simulink model "xi3_flatness"  (R2017b)
settings: Solver=VariableStepAuto  StartTime=0.0  StopTime=18  RelTol=1e-12
libraries: simulink x1
settings Model: Creator=chenjiasheng  LastModifiedBy=chenjiasheng

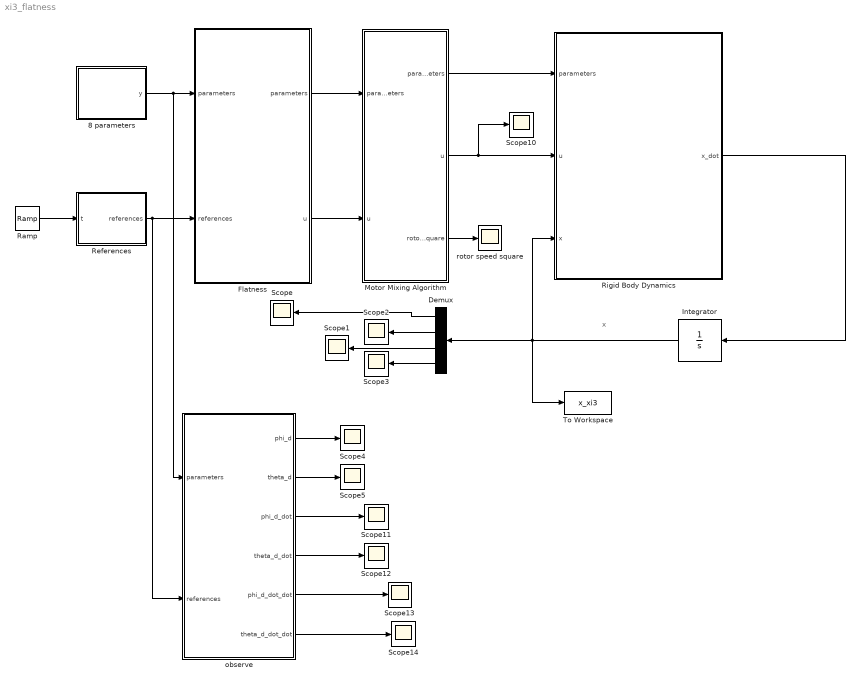
== system xi3_flatness ==
  note: x
  8 parameters : MATLAB Function  TreatAsAtomicUnit=on
  Demux : Demux
  Flatness : MATLAB Function  TreatAsAtomicUnit=on
  Integrator : Integrator  InitialCondition=x_xi2(end,:)  ContinuousStateAttributes='x'
  Motor Mixing Algorithm : MATLAB Function  TreatAsAtomicUnit=on
  Ramp : simulink/Sources/Ramp  slope=1  start=0  X0=0
  References : MATLAB Function  TreatAsAtomicUnit=on
  Rigid Body Dynamics : MATLAB Function  TreatAsAtomicUnit=on
  Scope{,1..5,10..14} (11 alike) : Scope
  To Workspace : ToWorkspace  VariableName=x_xi3  SampleTime=0.01
  observe : MATLAB Function  TreatAsAtomicUnit=on
  rotor speed square : Scope
  wires:
  Rigid Body Dynamics/1(x_dot) -> Integrator/1
  Motor Mixing Algorithm/3(rotor_speed_square) -> rotor speed square/1
  Motor Mixing Algorithm/1(parameters) -> Rigid Body Dynamics/1(parameters)
  Integrator/1 -> To Workspace/1, Demux/1, Rigid Body Dynamics/3(x)
  Motor Mixing Algorithm/2(u) -> Scope10/1, Rigid Body Dynamics/2(u)
  Ramp/1 -> References/1(t)
  Flatness/1(parameters) -> Motor Mixing Algorithm/1("parameters ")
  Flatness/2(u) -> Motor Mixing Algorithm/2("u ")
  References/1(references) -> Flatness/2(references), observe/2(references)
  8 parameters/1(y) -> Flatness/1("parameters "), observe/1(parameters)
  Demux/1 -> Scope/1
  Demux/3 -> Scope1/1
  Demux/2 -> Scope2/1
  Demux/4 -> Scope3/1
  observe/3(phi_d_dot) -> Scope11/1
  observe/4(theta_d_dot) -> Scope12/1
  observe/5(phi_d_dot_dot) -> Scope13/1
  observe/6(theta_d_dot_dot) -> Scope14/1
  observe/1(phi_d) -> Scope4/1
  observe/2(theta_d) -> Scope5/1

== matlab function xi3_flatness/Flatness ==
  data: parameters input; parameters output; references input; u output
function [parameters, u] = fcn(parameters,references)
% allocate input
m=parameters(1);
g=parameters(2);
M=diag(parameters(3:5));
r_d=references(1:3) ;          % reference's positions
r_d_dot=references(4:6);       % reference's velocities
a_d=references(7:9) ;          % reference's accelerations
a_d_dot=references(10:12);     % jerk
a_d_dot_dot=references(13:15); % snap
psi_d=references(16);          % reference's yaw angle 
psi_d_dot=references(17);
psi_d_dot_dot=references(18);

%% define some variables to make your life easier (f is not artifically defined)
f=m*sqrt(a_d(1)^2+a_d(2)^2+(g+a_d(3))^2);    % f is  the 1st element of input u
C=a_d(1)*cos(psi_d)+a_d(2)*sin(psi_d);      %
D=g+a_d(3);                                 %
A=a_d(1)*sin(psi_d)-a_d(2)*cos(psi_d);      %
B=sqrt(C^2+D^2);                            %
A_dot=sin(psi_d)*a_d_dot(1)-cos(psi_d)*a_d_dot(2)+C*psi_d_dot;                                   %
C_dot=cos(psi_d)*a_d_dot(1)+sin(psi_d)*a_d_dot(2)-A*psi_d_dot;                                   %
D_dot=a_d_dot(3);                                                                                %
B_dot=(C*C_dot+D*D_dot)/B;  
fbmsd=2*a_d(1)*a_d_dot(1)+2*a_d(2)*a_d_dot(2)+2*(g+a_d(3))*a_d_dot(3);   % f by m square dot
%% phi_d, theta_d
phi_d=asin(A*m/f) ;
if C>0
theta_d=acos(D/B) ;
else
theta_d=-acos(D/B) ;
end
%% phi_d_dot, theta_d_dot
phi_d_dot=(sin(psi_d)*(f/m)^2-A*a_d(1))/((f/m)^2*B)*a_d_dot(1) + (-cos(psi_d)*(f/m)^2-A*a_d(2))/((f/m)^2*B)*a_d_dot(2) + (-A*D)/((f/m)^2*B)*a_d_dot(3) + C/B*psi_d_dot;
theta_d_dot=(cos(psi_d)*D*a_d_dot(1)+sin(psi_d)*D*a_d_dot(2)-C*a_d_dot(3)-A*D*psi_d_dot)/B^2   ;

%% phi_d_dot_dot, theta_d_dot_dot
monster11=(cos(psi_d)*psi_d_dot*(f/m)^2+sin(psi_d)*fbmsd-(A_dot*a_d(1)+A*a_d_dot(1)))*a_d_dot(1)+(sin(psi_d)*(f/m)^2-A*a_d(1))*a_d_dot_dot(1);
monster12=(-sin(psi_d)*psi_d_dot*(f/m)^2+cos(psi_d)*fbmsd+A_dot*a_d(2)+A*a_d_dot(2))*a_d_dot(2)+(cos(psi_d)*(f/m)^2+A*a_d(2))*a_d_dot_dot(2);
monster13=(A_dot*D+A*D_dot)*a_d_dot(3)+A*D*a_d_dot_dot(3);
monster1=monster11-monster12-monster13;
phi_d_dot_dot=(monster1-(B*phi_d_dot-C*psi_d_dot)*fbmsd)/((f/m)^2*B) + (C_dot*psi_d_dot+C*psi_d_dot_dot-B_dot*phi_d_dot)/B;
monster21=(-sin(psi_d)*psi_d_dot*D+cos(psi_d)*D_dot)*a_d_dot(1)+cos(psi_d)*D*a_d_dot_dot(1);
monster22=(cos(psi_d)*psi_d_dot*D+sin(psi_d)*D_dot)*a_d_dot(2)+sin(psi_d)*D*a_d_dot_dot(2);
monster23= C_dot*a_d_dot(3)+C*a_d_dot_dot(3);
monster24=(A_dot*D+A*D_dot)*psi_d_dot+A*D*psi_d_dot_dot;
monster2= monster21+monster22-monster23-monster24;
theta_d_dot_dot=monster2/B^2-2*theta_d_dot*B_dot/B;

%% omegab, omegab_dot
Lnb=[1 0           -sin(theta_d);
     0 cos(phi_d)  sin(phi_d)*cos(theta_d);
     0 -sin(phi_d) cos(phi_d)*cos(theta_d)];
omegab=Lnb*[phi_d_dot;theta_d_dot;psi_d_dot];
omegab_dot=Lnb*[phi_d_dot_dot;theta_d_dot_dot;psi_d_dot_dot]+[-cos(theta_d)            0                        0;
                                                              -sin(phi_d)*sin(theta_d) cos(phi_d)*cos(theta_d)  -sin(phi_d);
                                                              -cos(phi_d)*sin(theta_d) -sin(phi_d)*cos(theta_d) -cos(phi_d)]*[theta_d_dot*psi_d_dot;phi_d_dot*psi_d_dot;phi_d_dot*theta_d_dot];

%% taub,u
taub=M*omegab_dot+cross(omegab,M*omegab);
u=[f;taub];
end

== matlab function xi3_flatness/8 parameters ==
  data: y output size=8
function y=fcn
%% specify parameters
m=0.468;
g=9.81;
Ix=4.856*10^(-3);
Iy=4.856*10^(-3);
Iz=8.801*10^(-3);
l=0.225;
k=2.980*10^-6;
c=1.140*10^-7;
%% output
y=[m;g;Ix;Iy;Iz;l;k;c] ;% output # 1-8
    
end

== matlab function xi3_flatness/observe ==
  data: parameters input; phi_d output; references input; theta_d output; phi_d_dot output; theta_d_dot output; phi_d_dot_dot output; theta_d_dot_dot output
function [phi_d,theta_d,phi_d_dot,theta_d_dot,phi_d_dot_dot,theta_d_dot_dot] = fcn(parameters,references)
% allocate input
m=parameters(1);
g=parameters(2);
M=diag(parameters(3:5));
r_d=references(1:3) ;          % reference's positions
r_d_dot=references(4:6);       % reference's velocities
a_d=references(7:9) ;          % reference's accelerations
a_d_dot=references(10:12);     % jerk
a_d_dot_dot=references(13:15); % snap
psi_d=references(16);          % reference's yaw angle 
psi_d_dot=references(17);
psi_d_dot_dot=references(18);

%% define some variables to make your life easier (f is not artifically defined)
f=m*sqrt(a_d(1)^2+a_d(2)^2+(g+a_d(3))^2);    % f is  the 1st element of input u
C=a_d(1)*cos(psi_d)+a_d(2)*sin(psi_d);      %
D=g+a_d(3);                                 %
A=a_d(1)*sin(psi_d)-a_d(2)*cos(psi_d);      %
B=sqrt(C^2+D^2);                            %
A_dot=sin(psi_d)*a_d_dot(1)-cos(psi_d)*a_d_dot(2)+C*psi_d_dot;                                   %   
C_dot=cos(psi_d)*a_d_dot(1)+sin(psi_d)*a_d_dot(2)-A*psi_d_dot;                                   %
D_dot=a_d_dot(3);                                                                                %
B_dot=(C*C_dot+D*D_dot)/B;
fbmsd=2*a_d(1)*a_d_dot(1)+2*a_d(2)*a_d_dot(2)+2*(g+a_d(3))*a_d_dot(3);   % f by m square dot
%% phi_d, theta_d
phi_d=asin(A*m/f) ;
if C>0
theta_d=acos(D/B) ;
else
theta_d=-acos(D/B) ;
end
%% phi_d_dot, theta_d_dot
phi_d_dot=(sin(psi_d)*(f/m)^2-A*a_d(1))/((f/m)^2*B)*a_d_dot(1) + (-cos(psi_d)*(f/m)^2-A*a_d(2))/((f/m)^2*B)*a_d_dot(2) + (-A*D)/((f/m)^2*B)*a_d_dot(3) + C/B*psi_d_dot;
theta_d_dot=(cos(psi_d)*D*a_d_dot(1)+sin(psi_d)*D*a_d_dot(2)-C*a_d_dot(3)-A*D*psi_d_dot)/B^2   ;

%% phi_d_dot_dot, theta_d_dot_dot
monster11=(cos(psi_d)*psi_d_dot*(f/m)^2+sin(psi_d)*fbmsd-(A_dot*a_d(1)+A*a_d_dot(1)))*a_d_dot(1)+(sin(psi_d)*(f/m)^2-A*a_d(1))*a_d_dot_dot(1);
monster12=(-sin(psi_d)*psi_d_dot*(f/m)^2+cos(psi_d)*fbmsd+A_dot*a_d(2)+A*a_d_dot(2))*a_d_dot(2)+(cos(psi_d)*(f/m)^2+A*a_d(2))*a_d_dot_dot(2);
monster13=(A_dot*D+A*D_dot)*a_d_dot(3)+A*D*a_d_dot_dot(3);
monster1=monster11-monster12-monster13;
phi_d_dot_dot=(monster1-(B*phi_d_dot-C*psi_d_dot)*fbmsd)/((f/m)^2*B) + (C_dot*psi_d_dot+C*psi_d_dot_dot-B_dot*phi_d_dot)/B;
monster21=(-sin(psi_d)*psi_d_dot*D+cos(psi_d)*D_dot)*a_d_dot(1)+cos(psi_d)*D*a_d_dot_dot(1);
monster22=(cos(psi_d)*psi_d_dot*D+sin(psi_d)*D_dot)*a_d_dot(2)+sin(psi_d)*D*a_d_dot_dot(2);
monster23= C_dot*a_d_dot(3)+C*a_d_dot_dot(3);
monster24=(A_dot*D+A*D_dot)*psi_d_dot+A*D*psi_d_dot_dot;
monster2= monster21+monster22-monster23-monster24;
theta_d_dot_dot=monster2/B^2-2*theta_d_dot*B_dot/B;

%% omegab, omegab_dot
Lnb=[1 0           -sin(theta_d);
     0 cos(phi_d)  sin(phi_d)*cos(theta_d);
     0 -sin(phi_d) cos(phi_d)*cos(theta_d)];
omegab=Lnb*[phi_d_dot;theta_d_dot;psi_d_dot];
omegab_dot=Lnb*[phi_d_dot_dot;theta_d_dot_dot;psi_d_dot_dot]+[-cos(theta_d)            0                        0;
                                                              -sin(phi_d)*sin(theta_d) cos(phi_d)*cos(theta_d)  -sin(phi_d);
                                                              -cos(phi_d)*sin(theta_d) -sin(phi_d)*cos(theta_d) -cos(phi_d)]*[theta_d_dot*psi_d_dot;phi_d_dot*psi_d_dot;phi_d_dot*theta_d_dot];

%% taub,u
taub=M*omegab_dot+cross(omegab,M*omegab);
u=[f;taub];
end

== matlab function xi3_flatness/References ==
  data: t input; references output size=18
function references = fcn(t)
%% specify your references here
g=9.81;
if t>=0 && t<2
r_desired=[0 0 0]'    ;              % reference's positions is not solved here
r_desired_dot=[0 0 0]'    ;          % reference's velocities is not solved here
r_desired_dot_dot=[0 0 0]'   ;       % reference's accelerations
r_desired_dot_dot_dot=[0 0 0]';      % jerk
r_desired_dot_dot_dot_dot=[0 0 0]' ; % snap
if t>=0 && t<1
psi_desired=pi/2-pi/4*t^2 ;                      % reference's yaw angle
psi_desired_dot=-pi/2*t;                  % reference's change rate of yaw angle       
psi_desired_dot_dot=-pi/2; 
else % t>=1 & t<2
psi_desired=pi/4*(t-2)^2 ;                      % reference's yaw angle
psi_desired_dot=pi/2*(t-2);                  % reference's change rate of yaw angle       
psi_desired_dot_dot=pi/2; 
end

elseif t>=2 && t<4  
if t>=2 && t<3
 r_desired=[0 0 0]'    ;              % reference's positions not solved here
 r_desired_dot=[0 0 0]'    ;          % reference's velocities not solved here
 r_desired_dot_dot=[0 0 -1]'   ;       % reference's accelerations
 r_desired_dot_dot_dot=[0 0 0]';      % jerk
 r_desired_dot_dot_dot_dot=[0 0 0]' ; % snap
else
 r_desired=[0 0 0]'    ;              % reference's positions 
 r_desired_dot=[0 0 0]'    ;          % reference's velocities 
 r_desired_dot_dot=[0 0 1]'   ;       % reference's accelerations
 r_desired_dot_dot_dot=[0 0 0]';      % jerk
 r_desired_dot_dot_dot_dot=[0 0 0]' ; % snap
end
 psi_desired=0 ;                      % reference's yaw angle
 psi_desired_dot=0 ;                  % reference's change rate of yaw angle       
 psi_desired_dot_dot=0;  
 
elseif t>=4 && t<6
tanalpha=0 ; % slope
if t>=4 && t<5
   [ax_d, az_d, ax_d_dot, az_d_dot, ax_d_dot_dot, az_d_dot_dot]=nest(t-4);
    ax_d=5/4*ax_d;                   az_d=5/4*az_d;
    ax_d_dot=5/4*ax_d_dot;           az_d_dot=5/4*az_d_dot;
    ax_d_dot_dot=5/4*ax_d_dot_dot;   az_d_dot_dot=5/4*az_d_dot_dot;
else % t>=5 && t<6
   [ax_d, az_d, ax_d_dot, az_d_dot, ax_d_dot_dot, az_d_dot_dot]=nest(t-5);
  ax_d=-5/4*ax_d;                 az_d=-5/4*az_d; % invert the direction for the sake of making end velocity zero
  ax_d_dot=-5/4*ax_d_dot;         az_d_dot=-5/4*az_d_dot;
  ax_d_dot_dot=-5/4*ax_d_dot_dot; az_d_dot_dot=-5/4*az_d_dot_dot;   
end  
 r_desired=[0 0 0]'    ;              % reference's positions is not solved here
 r_desired_dot=[0 0 0]'    ;          % reference's velocities is not solved here
 r_desired_dot_dot=[ax_d 0 az_d]'   ;       % reference's accelerations
 r_desired_dot_dot_dot=[ax_d_dot 0 az_d_dot]';      % jerk
 r_desired_dot_dot_dot_dot=[ax_d_dot_dot 0 az_d_dot_dot]' ; % snap
 psi_desired=0 ;                      % reference's yaw angle
 psi_desired_dot=0 ;                  % reference's change rate of yaw angle       
 psi_desired_dot_dot=0;
 
elseif t>=6 && t<8
r_desired=[0 0 0]'    ;              % reference's positions is not solved here
r_desired_dot=[0 0 0]'    ;          % reference's velocities is not solved here
r_desired_dot_dot=[0 0 0]'   ;       % reference's accelerations
r_desired_dot_dot_dot=[0 0 0]';      % jerk
r_desired_dot_dot_dot_dot=[0 0 0]' ; % snap
if t>=6 && t<7
psi_desired=pi/4*(t-6)^2 ;                      % reference's yaw angle
psi_desired_dot=pi/2*(t-6);                  % reference's change rate of yaw angle       
psi_desired_dot_dot=pi/2; 
else % t>=7 && t<8
psi_desired=-pi/4*(t-8)^2+pi/2 ;                      % reference's yaw angle
psi_desired_dot=-pi/2*(t-8);                  % reference's change rate of yaw angle       
psi_desired_dot_dot=-pi/2; 
end

elseif t>=8 && t<10
tanalpha=5/11 ; % slope
if t>=8 && t<9
   [ax_d, az_d, ax_d_dot, az_d_dot, ax_d_dot_dot, az_d_dot_dot]=nest(t-8);
    ax_d=-1102/329*ax_d;                   az_d=-1102/329*az_d;
    ax_d_dot=-1102/329*ax_d_dot;           az_d_dot=-1102/329*az_d_dot;
    ax_d_dot_dot=-1102/329*ax_d_dot_dot;   az_d_dot_dot=-1102/329*az_d_dot_dot;
else % t>=9 && t<10
   [ax_d, az_d, ax_d_dot, az_d_dot, ax_d_dot_dot, az_d_dot_dot]=nest(t-9);
  ax_d=1102/329*ax_d;                 az_d=1102/329*az_d; % invert the direction for the sake of making end velocity zero
  ax_d_dot=1102/329*ax_d_dot;         az_d_dot=1102/329*az_d_dot;
  ax_d_dot_dot=1102/329*ax_d_dot_dot; az_d_dot_dot=1102/329*az_d_dot_dot;   
end  
 r_desired=[0 0 0]'    ;              % reference's positions is not solved here
 r_desired_dot=[0 0 0]'    ;          % reference's velocities is not solved here
 r_desired_dot_dot=[ax_d 0 az_d]'   ;       % reference's accelerations
 r_desired_dot_dot_dot=[ax_d_dot 0 az_d_dot]';      % jerk
 r_desired_dot_dot_dot_dot=[ax_d_dot_dot 0 az_d_dot_dot]' ; % snap
 psi_desired=pi/2 ;                      % reference's yaw angle
 psi_desired_dot=0 ;                  % reference's change rate of yaw angle       
 psi_desired_dot_dot=0;
 
elseif t>=10 && t<12
r_desired=[0 0 0]'    ;              % reference's positions is not solved here
r_desired_dot=[0 0 0]'    ;          % reference's velocities is not solved here
r_desired_dot_dot=[0 0 0]'   ;       % reference's accelerations
r_desired_dot_dot_dot=[0 0 0]';      % jerk
r_desired_dot_dot_dot_dot=[0 0 0]' ; % snap
if t>=10 && t<11
psi_desired=pi/2-pi/4*(t-10)^2 ;                      % reference's yaw angle
psi_desired_dot=-pi/2*(t-10);                  % reference's change rate of yaw angle       
psi_desired_dot_dot=-pi/2; 
else % t>=11 & t<12
psi_desired=pi/4*(t-12)^2 ;                      % reference's yaw angle
psi_desired_dot=pi/2*(t-12);                  % reference's change rate of yaw angle       
psi_desired_dot_dot=pi/2; 
end

elseif t>=12 && t<14
tanalpha=0 ; % slope
if t>=12 && t<13
   [ax_d, az_d, ax_d_dot, az_d_dot, ax_d_dot_dot, az_d_dot_dot]=nest(t-12);
    ax_d=3.5*ax_d;                   az_d=3.5*az_d;
    ax_d_dot=3.5*ax_d_dot;           az_d_dot=3.5*az_d_dot;
    ax_d_dot_dot=3.5*ax_d_dot_dot;   az_d_dot_dot=3.5*az_d_dot_dot;
else % t>=13 && t<14
   [ax_d, az_d, ax_d_dot, az_d_dot, ax_d_dot_dot, az_d_dot_dot]=nest(t-13);
  ax_d=-3.5*ax_d;                 az_d=-3.5*az_d; % invert the direction for the sake of making end velocity zero
  ax_d_dot=-3.5*ax_d_dot;         az_d_dot=-3.5*az_d_dot;
  ax_d_dot_dot=-3.5*ax_d_dot_dot; az_d_dot_dot=-3.5*az_d_dot_dot;   
end  
 r_desired=[0 0 0]'    ;              % reference's positions is not solved here
 r_desired_dot=[0 0 0]'    ;          % reference's velocities is not solved here
 r_desired_dot_dot=[ax_d 0 az_d]'   ;       % reference's accelerations
 r_desired_dot_dot_dot=[ax_d_dot 0 az_d_dot]';      % jerk
 r_desired_dot_dot_dot_dot=[ax_d_dot_dot 0 az_d_dot_dot]' ; % snap
 psi_desired=0 ;                      % reference's yaw angle
 psi_desired_dot=0 ;                  % reference's change rate of yaw angle       
 psi_desired_dot_dot=0;
 
elseif t>=14 && t<16
r_desired=[0 0 0]'    ;              % reference's positions is not solved here
r_desired_dot=[0 0 0]'    ;          % reference's velocities is not solved here
r_desired_dot_dot=[0 0 0]'   ;       % reference's accelerations
r_desired_dot_dot_dot=[0 0 0]';      % jerk
r_desired_dot_dot_dot_dot=[0 0 0]' ; % snap
if t>=14 && t<15
psi_desired=pi/4*(t-14)^2 ;                      % reference's yaw angle
psi_desired_dot=pi/2*(t-14);                  % reference's change rate of yaw angle       
psi_desired_dot_dot=pi/2; 
else % t>=15 && t<16
psi_desired=-pi/4*(t-16)^2+pi/2 ;                      % reference's yaw angle
psi_desired_dot=-pi/2*(t-16);                  % reference's change rate of yaw angle       
psi_desired_dot_dot=-pi/2; 
end

else
tanalpha=5 ; % slope
if t>=16 && t<17
   [ax_d, az_d, ax_d_dot, az_d_dot, ax_d_dot_dot, az_d_dot_dot]=nest(t-16);
    ax_d=1500/2168*ax_d;                   az_d=1500/2168*az_d;
    ax_d_dot=1500/2168*ax_d_dot;           az_d_dot=1500/2168*az_d_dot;
    ax_d_dot_dot=1500/2168*ax_d_dot_dot;   az_d_dot_dot=1500/2168*az_d_dot_dot;
else % t>=17 && t<18
   [ax_d, az_d, ax_d_dot, az_d_dot, ax_d_dot_dot, az_d_dot_dot]=nest(t-17);
  ax_d=-1500/2168*ax_d;                 az_d=-1500/2168*az_d; % invert the direction for the sake of making end velocity zero
  ax_d_dot=-1500/2168*ax_d_dot;         az_d_dot=-1500/2168*az_d_dot;
  ax_d_dot_dot=-1500/2168*ax_d_dot_dot; az_d_dot_dot=-1500/2168*az_d_dot_dot;   
end  
 r_desired=[0 0 0]'    ;              % reference's positions is not solved here
 r_desired_dot=[0 0 0]'    ;          % reference's velocities is not solved here
 r_desired_dot_dot=[ax_d 0 az_d]'   ;       % reference's accelerations
 r_desired_dot_dot_dot=[ax_d_dot 0 az_d_dot]';      % jerk
 r_desired_dot_dot_dot_dot=[ax_d_dot_dot 0 az_d_dot_dot]' ; % snap
 psi_desired=pi/2 ;                      % reference's yaw angle
 psi_desired_dot=0 ;                  % reference's change rate of yaw angle       
 psi_desired_dot_dot=0;
end

references=[r_desired;                 %  1-3
            r_desired_dot;             %  4-6
            r_desired_dot_dot;         %  7-9
            r_desired_dot_dot_dot;     %  10-12
            r_desired_dot_dot_dot_dot; %  13-15
            psi_desired;               %  16
            psi_desired_dot;           %  17
            psi_desired_dot_dot];      %  18
        
  function   [axn, azn, axn_dot, azn_dot, axn_dot_dot, azn_dot_dot]=nest(tn)
        if tn>=0 && tn<1/4
        angle=pi/6*tn^2;               angle_dot=pi/3*tn;           angle_dot_dot=pi/3;
        elseif tn>=1/4 && tn<3/4
        angle=-pi/6*(tn-1/2)^2+pi/48;  angle_dot=-pi/3*(tn-1/2);    angle_dot_dot=-pi/3;
        else 
        angle=pi/6*(tn-1)^2;           angle_dot=pi/3*(tn-1);       angle_dot_dot=pi/3;
        end
     axn=g*tan(angle)/(1-tanalpha*tan(angle));
     azn=tanalpha*axn;
     axn_dot=g*(1+tan(angle)^2)*angle_dot/(1-tanalpha*tan(angle))^2;
     azn_dot=tanalpha*axn_dot;
     axn_dot_dot=g*(1+tan(angle)^2)*(2*angle_dot^2*(tan(angle)+tanalpha)+angle_dot_dot*(1-tanalpha*tan(angle)))/(1-tanalpha*tan(angle))^3;
     azn_dot_dot=tanalpha*axn_dot_dot;
  end


end       
%% sources
%% -------- a horizontal circle with radius of 3 m-------------------------------
% r_desired=[3*cos(t) 3*sin(t) 0]'    ;             % reference's positions
% r_desired_dot=[-3*sin(t) 3*cos(t) 0]'    ;        % reference's velocities
% r_desired_dot_dot=[-3*cos(t) -3*sin(t) 0]'   ;    % reference's accelerations
% r_desired_dot_dot_dot=[3*sin(t) -3*cos(t) 0]';    % jerk
% r_desired_dot_dot_dot_dot=[3*cos(t) 3*sin(t) 0]' ;% snap
% psi_desired=0 ;                % reference's yaw angle
% psi_desired_dot=0 ;            % reference's change rate of yaw angle    
% psi_desired_dot_dot=0;
% [3 0 0,0 3 0,0 -acos(9.81/sqrt(9+9.81^2)) 0,3/sqrt(9+9.81^2) 0 0] % initial condition
%% -------- a vertiacal circle with radius of 3 m-------------------------------
% r_desired=[0 3*sin(t) -3*cos(t)]'    ;             % reference's positions
% r_desired_dot=[0 3*cos(t) 3*sin(t)]'    ;        % reference's velocities
% r_desired_dot_dot=[0 -3*sin(t) 3*cos(t)]'   ;    % reference's accelerations
% r_desired_dot_dot_dot=[0 -3*cos(t) -3*sin(t)]';    % jerk
% r_desired_dot_dot_dot_dot=[0 3*sin(t) -3*cos(t)]' ;% snap
% psi_desired=0 ;                % reference's yaw angle
% psi_desired_dot=0 ;            % reference's change rate of yaw angle    
% psi_desired_dot_dot=0;
%% ------------------a horizontal straight line--------------------------
% g=9.81;
%  if t>=0 & t<1 
%     theta_d=pi/6*t^2 ;           theta_d_dot=pi/3*t ;      theta_d_dot_dot=pi/3;
%  elseif t>=1 & t<3
%     theta_d=-pi/6*(t-2)^2+pi/3 ; theta_d_dot=-pi/3*(t-2) ; theta_d_dot_dot=-pi/3;
%  elseif t>=3 & t<4
%     theta_d=pi/6*(t-4)^2 ;       theta_d_dot=pi/3*(t-4) ;  theta_d_dot_dot=pi/3;
%  elseif t>=4 & t<5
%     theta_d=-pi/6*(t-4)^2 ;      theta_d_dot=-pi/3*(t-4) ; theta_d_dot_dot=-pi/3;
%  elseif t>=5 & t<7
%     theta_d=pi/6*(t-6)^2-pi/3 ;  theta_d_dot=pi/3*(t-6) ;  theta_d_dot_dot=pi/3;
%  else 
%     theta_d=-pi/6*(t-8)^2 ;      theta_d_dot=-pi/3*(t-8);  theta_d_dot_dot=-pi/3;
%  end
%  r_desired=[0 0 0]'    ;              % reference's positions is not solved here
%  r_desired_dot=[0 0 0]'    ;          % reference's velocities is not solved here
%  r_desired_dot_dot=[1/100*g*tan(theta_d) 0 0]'   ;       % reference's accelerations
%  r_desired_dot_dot_dot=[1/100*g*(1+tan(theta_d)^2)*theta_d_dot 0 0]';      % jerk
%  r_desired_dot_dot_dot_dot=[1/100*g*(1+tan(theta_d)^2)*(2*tan(theta_d)*theta_d_dot^2+theta_d_dot_dot) 0 0]' ; % snap
%  psi_desired=0 ;                      % reference's yaw angle
%  psi_desired_dot=0 ;                  % reference's change rate of yaw angle       
%  psi_desired_dot_dot=0;
%% -----------a vertical straight line------------------
% if t<1
%  r_desired=[0 0 t^2]'    ;              % reference's positions 
%  r_desired_dot=[0 0 2*t]'    ;          % reference's velocities
%  r_desired_dot_dot=[0 0 2]'   ;       % reference's accelerations
%  r_desired_dot_dot_dot=[0 0 0]';      % jerk
%  r_desired_dot_dot_dot_dot=[0 0 0]' ; % snap
% else
%  r_desired=[0 0 -(t-2)^2+2]'    ;              % reference's positions 
%  r_desired_dot=[0 0 -2*(t-2)]'    ;          % reference's velocities 
%  r_desired_dot_dot=[0 0 -2]'   ;       % reference's accelerations
%  r_desired_dot_dot_dot=[0 0 0]';      % jerk
%  r_desired_dot_dot_dot_dot=[0 0 0]' ; % snap
% end
%  psi_desired=0 ;                      % reference's yaw angle
%  psi_desired_dot=0 ;                  % reference's change rate of yaw angle       
%  psi_desired_dot_dot=0;
%% --------W------------------------------------
% g=9.81;
% if t>=0 & t<8
%  if t>=0 & t<1 
%     theta_d=pi/6*t^2 ;           theta_d_dot=pi/3*t ;      theta_d_dot_dot=pi/3;
%  elseif t>=1 & t<3
%     theta_d=-pi/6*(t-2)^2+pi/3 ; theta_d_dot=-pi/3*(t-2) ; theta_d_dot_dot=-pi/3;
%  elseif t>=3 & t<4
%     theta_d=pi/6*(t-4)^2 ;       theta_d_dot=pi/3*(t-4) ;  theta_d_dot_dot=pi/3;
%  elseif t>=4 & t<5
%     theta_d=-pi/6*(t-4)^2 ;      theta_d_dot=-pi/3*(t-4) ; theta_d_dot_dot=-pi/3;
%  elseif t>=5 & t<7
%     theta_d=pi/6*(t-6)^2-pi/3 ;  theta_d_dot=pi/3*(t-6) ;  theta_d_dot_dot=pi/3;
%  else 
%     theta_d=-pi/6*(t-8)^2 ;      theta_d_dot=-pi/3*(t-8);  theta_d_dot_dot=-pi/3;
%  end
%  r_desired=[0 0 0]'    ;              % reference's positions is not solved here
%  r_desired_dot=[0 0 0]'    ;          % reference's velocities is not solved here
%  r_desired_dot_dot=[1/200*g*tan(theta_d) -sqrt(3)/200*g*tan(theta_d) 0]'   ;       % reference's accelerations
%  r_desired_dot_dot_dot=[1/200*g*(1+tan(theta_d)^2)*theta_d_dot -sqrt(3)/200*g*(1+tan(theta_d)^2)*theta_d_dot 0]';      % jerk
%  r_desired_dot_dot_dot_dot=[1/200*g*(1+tan(theta_d)^2)*(2*tan(theta_d)*theta_d_dot^2+theta_d_dot_dot) -sqrt(3)/200*g*(1+tan(theta_d)^2)*(2*tan(theta_d)*theta_d_dot^2+theta_d_dot_dot) 0]' ; % snap
%  psi_desired=-pi/3 ;                      % reference's yaw angle
%  psi_desired_dot=0 ;                  % reference's change rate of yaw angle       
%  psi_desired_dot_dot=0;
%  
% elseif t>=8 & t<10 
% r_desired=[0 0 0]'    ;              % reference's positions 
% r_desired_dot=[0 0 0]'    ;          % reference's velocities
% r_desired_dot_dot=[0 0 0]'   ;       % reference's accelerations
% r_desired_dot_dot_dot=[0 0 0]';      % jerk
% r_desired_dot_dot_dot_dot=[0 0 0]' ; % snap
% if t>=8 & t<9
% psi_desired=-pi/3+pi/3*(t-8)^2 ;                      % reference's yaw angle
% psi_desired_dot=pi*2/3*(t-8);                  % reference's change rate of yaw angle       
% psi_desired_dot_dot=pi*2/3; 
% else
% psi_desired=-pi/3*(t-10)^2+pi/3 ;                      % reference's yaw angle
% psi_desired_dot=-pi*2/3*(t-10);                  % reference's change rate of yaw angle       
% psi_desired_dot_dot=-pi*2/3; 
% end
% 
% elseif t>=10 & t<18
%   if t>=10 & t<11 
%     theta_d=pi/6*(t-10)^2 ;           theta_d_dot=pi/3*(t-10) ;      theta_d_dot_dot=pi/3;
%  elseif t>=11 & t<13
%     theta_d=-pi/6*(t-12)^2+pi/3 ; theta_d_dot=-pi/3*(t-12) ; theta_d_dot_dot=-pi/3;
%  elseif t>=13 & t<14
%     theta_d=pi/6*(t-14)^2 ;       theta_d_dot=pi/3*(t-14) ;  theta_d_dot_dot=pi/3;
%  elseif t>=14 & t<15
%     theta_d=-pi/6*(t-14)^2 ;      theta_d_dot=-pi/3*(t-14) ; theta_d_dot_dot=-pi/3;
%  elseif t>=15 & t<17
%     theta_d=pi/6*(t-16)^2-pi/3 ;  theta_d_dot=pi/3*(t-16) ;  theta_d_dot_dot=pi/3;
%  else 
%     theta_d=-pi/6*(t-18)^2 ;      theta_d_dot=-pi/3*(t-18);  theta_d_dot_dot=-pi/3;
%  end
%  r_desired=[0 0 0]'    ;              % reference's positions is not solved here
%  r_desired_dot=[0 0 0]'    ;          % reference's velocities is not solved here
%  r_desired_dot_dot=[1/200*g*tan(theta_d) sqrt(3)/200*g*tan(theta_d) 0]'   ;       % reference's accelerations
%  r_desired_dot_dot_dot=[1/200*g*(1+tan(theta_d)^2)*theta_d_dot sqrt(3)/200*g*(1+tan(theta_d)^2)*theta_d_dot 0]';      % jerk
%  r_desired_dot_dot_dot_dot=[1/200*g*(1+tan(theta_d)^2)*(2*tan(theta_d)*theta_d_dot^2+theta_d_dot_dot) sqrt(3)/200*g*(1+tan(theta_d)^2)*(2*tan(theta_d)*theta_d_dot^2+theta_d_dot_dot) 0]' ; % snap
%  psi_desired=pi/3 ;                      % reference's yaw angle
%  psi_desired_dot=0 ;                  % reference's change rate of yaw angle       
%  psi_desired_dot_dot=0;  
%  
% elseif t>=18 & t<20
% r_desired=[0 0 0]'    ;              % reference's positions 
% r_desired_dot=[0 0 0]'    ;          % reference's velocities
% r_desired_dot_dot=[0 0 0]'   ;       % reference's accelerations
% r_desired_dot_dot_dot=[0 0 0]';      % jerk
% r_desired_dot_dot_dot_dot=[0 0 0]' ; % snap
% if t>=18 & t<19
% psi_desired=pi/3-pi/3*(t-18)^2 ;                      % reference's yaw angle
% psi_desired_dot=-pi*2/3*(t-18);                  % reference's change rate of yaw angle       
% psi_desired_dot_dot=-pi*2/3; 
% else
% psi_desired=pi/3*(t-20)^2-pi/3 ;                      % reference's yaw angle
% psi_desired_dot=pi*2/3*(t-20);                  % reference's change rate of yaw angle       
% psi_desired_dot_dot=pi*2/3; 
% end
% 
% elseif t>=20 & t<28
%  if t>=20 & t<21 
%     theta_d=pi/6*(t-20)^2 ;           theta_d_dot=pi/3*(t-20) ;      theta_d_dot_dot=pi/3;
%  elseif t>=21 & t<23
%     theta_d=-pi/6*(t-22)^2+pi/3 ; theta_d_dot=-pi/3*(t-22) ; theta_d_dot_dot=-pi/3;
%  elseif t>=23 & t<24
%     theta_d=pi/6*(t-24)^2 ;       theta_d_dot=pi/3*(t-24) ;  theta_d_dot_dot=pi/3;
%  elseif t>=24 & t<25
%     theta_d=-pi/6*(t-24)^2 ;      theta_d_dot=-pi/3*(t-24) ; theta_d_dot_dot=-pi/3;
%  elseif t>=25 & t<27
%     theta_d=pi/6*(t-26)^2-pi/3 ;  theta_d_dot=pi/3*(t-26) ;  theta_d_dot_dot=pi/3;
%  else 
%     theta_d=-pi/6*(t-28)^2 ;      theta_d_dot=-pi/3*(t-28);  theta_d_dot_dot=-pi/3;
%  end
%  r_desired=[0 0 0]'    ;              % reference's positions is not solved here
%  r_desired_dot=[0 0 0]'    ;          % reference's velocities is not solved here
%  r_desired_dot_dot=[1/200*g*tan(theta_d) -sqrt(3)/200*g*tan(theta_d) 0]'   ;       % reference's accelerations
%  r_desired_dot_dot_dot=[1/200*g*(1+tan(theta_d)^2)*theta_d_dot -sqrt(3)/200*g*(1+tan(theta_d)^2)*theta_d_dot 0]';      % jerk
%  r_desired_dot_dot_dot_dot=[1/200*g*(1+tan(theta_d)^2)*(2*tan(theta_d)*theta_d_dot^2+theta_d_dot_dot) -sqrt(3)/200*g*(1+tan(theta_d)^2)*(2*tan(theta_d)*theta_d_dot^2+theta_d_dot_dot) 0]' ; % snap
%  psi_desired=-pi/3 ;                      % reference's yaw angle
%  psi_desired_dot=0 ;                      % reference's change rate of yaw angle       
%  psi_desired_dot_dot=0; 
%  
% elseif t>=28 & t<30
% r_desired=[0 0 0]'    ;              % reference's positions 
% r_desired_dot=[0 0 0]'    ;          % reference's velocities
% r_desired_dot_dot=[0 0 0]'   ;       % reference's accelerations
% r_desired_dot_dot_dot=[0 0 0]';      % jerk
% r_desired_dot_dot_dot_dot=[0 0 0]' ; % snap
% if t>=28 & t<29
% psi_desired=-pi/3+pi/3*(t-28)^2 ;                      % reference's yaw angle
% psi_desired_dot=pi*2/3*(t-28);                  % reference's change rate of yaw angle       
% psi_desired_dot_dot=pi*2/3; 
% else
% psi_desired=-pi/3*(t-30)^2+pi/3 ;                      % reference's yaw angle
% psi_desired_dot=-pi*2/3*(t-30);                  % reference's change rate of yaw angle       
% psi_desired_dot_dot=-pi*2/3; 
% end
% 
% else
% if t>=30 & t<31 
%     theta_d=pi/6*(t-30)^2 ;           theta_d_dot=pi/3*(t-30) ;      theta_d_dot_dot=pi/3;
%  elseif t>=31 & t<33
%     theta_d=-pi/6*(t-32)^2+pi/3 ; theta_d_dot=-pi/3*(t-32) ; theta_d_dot_dot=-pi/3;
%  elseif t>=33 & t<34
%     theta_d=pi/6*(t-34)^2 ;       theta_d_dot=pi/3*(t-34) ;  theta_d_dot_dot=pi/3;
%  elseif t>=34 & t<35
%     theta_d=-pi/6*(t-34)^2 ;      theta_d_dot=-pi/3*(t-34) ; theta_d_dot_dot=-pi/3;
%  elseif t>=35 & t<37
%     theta_d=pi/6*(t-36)^2-pi/3 ;  theta_d_dot=pi/3*(t-36) ;  theta_d_dot_dot=pi/3;
%  else 
%     theta_d=-pi/6*(t-38)^2 ;      theta_d_dot=-pi/3*(t-38);  theta_d_dot_dot=-pi/3;
%  end
%  r_desired=[0 0 0]'    ;              % reference's positions is not solved here
%  r_desired_dot=[0 0 0]'    ;          % reference's velocities is not solved here
%  r_desired_dot_dot=[1/200*g*tan(theta_d) sqrt(3)/200*g*tan(theta_d) 0]'   ;       % reference's accelerations
%  r_desired_dot_dot_dot=[1/200*g*(1+tan(theta_d)^2)*theta_d_dot sqrt(3)/200*g*(1+tan(theta_d)^2)*theta_d_dot 0]';      % jerk
%  r_desired_dot_dot_dot_dot=[1/200*g*(1+tan(theta_d)^2)*(2*tan(theta_d)*theta_d_dot^2+theta_d_dot_dot) sqrt(3)/200*g*(1+tan(theta_d)^2)*(2*tan(theta_d)*theta_d_dot^2+theta_d_dot_dot) 0]' ; % snap
%  psi_desired=pi/3 ;                      % reference's yaw angle
%  psi_desired_dot=0 ;                  % reference's change rate of yaw angle       
%  psi_desired_dot_dot=0;  
%
% end
%% ------------xi hu da xue---------
% g=9.81;
% if t>=0 & t<8
%  if t>=0 & t<1 
%     theta_d=pi/6*t^2 ;           theta_d_dot=pi/3*t ;      theta_d_dot_dot=pi/3;
%  elseif t>=1 & t<3
%     theta_d=-pi/6*(t-2)^2+pi/3 ; theta_d_dot=-pi/3*(t-2) ; theta_d_dot_dot=-pi/3;
%  elseif t>=3 & t<4
%     theta_d=pi/6*(t-4)^2 ;       theta_d_dot=pi/3*(t-4) ;  theta_d_dot_dot=pi/3;
%  elseif t>=4 & t<5
%     theta_d=-pi/6*(t-4)^2 ;      theta_d_dot=-pi/3*(t-4) ; theta_d_dot_dot=-pi/3;
%  elseif t>=5 & t<7
%     theta_d=pi/6*(t-6)^2-pi/3 ;  theta_d_dot=pi/3*(t-6) ;  theta_d_dot_dot=pi/3;
%  else % t>=7 & t<8
%     theta_d=-pi/6*(t-8)^2 ;      theta_d_dot=-pi/3*(t-8);  theta_d_dot_dot=-pi/3;
%  end
%  r_desired=[0 0 0]'    ;              % reference's positions is not solved here
%  r_desired_dot=[0 0 0]'    ;          % reference's velocities is not solved here
%  r_desired_dot_dot=[1/100*g*tan(theta_d) 0 0]'   ;       % reference's accelerations
%  r_desired_dot_dot_dot=[1/100*g*(1+tan(theta_d)^2)*theta_d_dot 0 0]';      % jerk
%  r_desired_dot_dot_dot_dot=[1/100*g*(1+tan(theta_d)^2)*(2*tan(theta_d)*theta_d_dot^2+theta_d_dot_dot) 0 0]' ; % snap
%  psi_desired=0 ;                      % reference's yaw angle
%  psi_desired_dot=0 ;                  % reference's change rate of yaw angle       
%  psi_desired_dot_dot=0;
%  
% elseif t>=8 & t<10
% r_desired=[0 0 0]'    ;              % reference's positions is not solved here
% r_desired_dot=[0 0 0]'    ;          % reference's velocities is not solved here
% r_desired_dot_dot=[0 0 0]'   ;       % reference's accelerations
% r_desired_dot_dot_dot=[0 0 0]';      % jerk
% r_desired_dot_dot_dot_dot=[0 0 0]' ; % snap
% if t>=8 & t<9
% psi_desired=pi/4*(t-8)^2 ;                      % reference's yaw angle
% psi_desired_dot=pi/2*(t-8);                  % reference's change rate of yaw angle       
% psi_desired_dot_dot=pi/2; 
% else % t>=9 & t<10
% psi_desired=-pi/4*(t-10)^2+pi/2 ;                      % reference's yaw angle
% psi_desired_dot=-pi/2*(t-10);                  % reference's change rate of yaw angle       
% psi_desired_dot_dot=-pi/2; 
% end
% 
% elseif t>=10 & t<12
% if t>=10 & t<11
%  r_desired=[0 0 -1/4*(t-10)^2]'    ;              % reference's positions 
%  r_desired_dot=[0 0 -1/2*(t-8)]'    ;          % reference's velocities
%  r_desired_dot_dot=[0 0 -1/2]'   ;       % reference's accelerations
%  r_desired_dot_dot_dot=[0 0 0]';      % jerk
%  r_desired_dot_dot_dot_dot=[0 0 0]' ; % snap
% else % t>=11 & t<12
%  r_desired=[0 0 1/4*(t-12)^2+1/2]'    ;              % reference's positions 
%  r_desired_dot=[0 0 1/2*(t-12)]'    ;          % reference's velocities 
%  r_desired_dot_dot=[0 0 1/2]'   ;       % reference's accelerations
%  r_desired_dot_dot_dot=[0 0 0]';      % jerk
%  r_desired_dot_dot_dot_dot=[0 0 0]' ; % snap
% end
%  psi_desired=pi/2;                      % reference's yaw angle
%  psi_desired_dot=0 ;                  % reference's change rate of yaw angle       
%  psi_desired_dot_dot=0;
%  
% elseif t>=12 & t<20
% if t>=12 & t<13 
%     phi_d=-pi/6*(t-12)^2 ;           phi_d_dot=-pi/3*(t-12) ;      phi_d_dot_dot=-pi/3;
%  elseif t>=13 & t<15
%     phi_d=pi/6*(t-14)^2-pi/3 ;       phi_d_dot=pi/3*(t-14) ;       phi_d_dot_dot=pi/3;
%  elseif t>=15 & t<16
%     phi_d=-pi/6*(t-16)^2 ;           phi_d_dot=-pi/3*(t-16) ;      phi_d_dot_dot=-pi/3;
%  elseif t>=16 & t<17
%     phi_d=pi/6*(t-16)^2 ;            phi_d_dot=pi/3*(t-16) ;       phi_d_dot_dot=pi/3;
%  elseif t>=17 & t<19
%     phi_d=-pi/6*(t-18)^2+pi/3 ;      phi_d_dot=-pi/3*(t-18) ;      phi_d_dot_dot=-pi/3;
%  else % t>=19 & t<20
%     phi_d=pi/6*(t-20)^2 ;            phi_d_dot=pi/3*(t-20);        phi_d_dot_dot=pi/3;
% end
%  r_desired=[0 0 0]'    ;              % reference's positions is not solved here
%  r_desired_dot=[0 0 0]'    ;          % reference's velocities is not solved here
%  r_desired_dot_dot=[1/100*g*tan(phi_d) 0 0]'   ;       % reference's accelerations
%  r_desired_dot_dot_dot=[1/100*g*(1+tan(phi_d)^2)*phi_d_dot 0 0]';      % jerk
%  r_desired_dot_dot_dot_dot=[1/100*g*(1+tan(phi_d)^2)*(2*tan(phi_d)*phi_d_dot^2+phi_d_dot_dot) 0 0]' ; % snap
%  psi_desired=pi/2 ;                      % reference's yaw angle
%  psi_desired_dot=0 ;                  % reference's change rate of yaw angle       
%  psi_desired_dot_dot=0;
%  
% elseif t>=20 & t<22
% r_desired=[0 0 0]'    ;              % reference's positions is not solved here
% r_desired_dot=[0 0 0]'    ;          % reference's velocities is not solved here
% r_desired_dot_dot=[0 0 0]'   ;       % reference's accelerations
% r_desired_dot_dot_dot=[0 0 0]';      % jerk
% r_desired_dot_dot_dot_dot=[0 0 0]' ; % snap
% if t>=20 & t<21
% psi_desired=pi/2-pi/4*(t-20)^2 ;                      % reference's yaw angle
% psi_desired_dot=-pi/2*(t-20);                  % reference's change rate of yaw angle       
% psi_desired_dot_dot=-pi/2; 
% else % t>=21 & t<22
% psi_desired=pi/4*(t-22)^2 ;                      % reference's yaw angle
% psi_desired_dot=pi/2*(t-22);                  % reference's change rate of yaw angle       
% psi_desired_dot_dot=pi/2; 
% end
% 
% else
% if t>=22 & t<23
%  r_desired=[0 0 -1/2*(t-22)^2-1/2]'    ;              % reference's positions 
%  r_desired_dot=[0 0 -(t-22)]'    ;          % reference's velocities
%  r_desired_dot_dot=[0 0 -1]'   ;       % reference's accelerations
%  r_desired_dot_dot_dot=[0 0 0]';      % jerk
%  r_desired_dot_dot_dot_dot=[0 0 0]' ; % snap
% else % t>=23 & t<24
%  r_desired=[0 0 1/2*(t-24)^2-3/2]'    ;              % reference's positions 
%  r_desired_dot=[0 0 (t-24)]'    ;          % reference's velocities 
%  r_desired_dot_dot=[0 0 1]'   ;       % reference's accelerations
%  r_desired_dot_dot_dot=[0 0 0]';      % jerk
%  r_desired_dot_dot_dot_dot=[0 0 0]' ; % snap
% end
%  psi_desired=0 ;                      % reference's yaw angle
%  psi_desired_dot=0 ;                  % reference's change rate of yaw angle       
%  psi_desired_dot_dot=0;
% 
% end

== matlab function xi3_flatness/Motor Mixing Algorithm ==
  data: parameters output; u output; parameters input size=8; u input size=4; rotor_speed_square output size=4
function [parameters,u,rotor_speed_square]=fcn(parameters,u)
l=parameters(6) ; 
k=parameters(7) ;
c=parameters(8) ;
rotor_speed_square=[1 0 -1  1;
                    1 1  0 -1;
                    1 0  1  1;
                    1 -1 0 -1]* [1/(4*k) 0         0         0;
                                0        1/(2*l*k) 0         0;
                                0        0         1/(2*l*k) 0;
                                0        0         0         1/(4*c)]*u ;
end
%% Motor dynamics
% rotor_speed=in(9:12)
% rotor_speed_square=rotor_speed.^2
%f_taux_tauy_tauz=[k 0   0   0;
%                  0 k*l 0   0;
%                  0 0   k*l 0;
%                  0 0   0   c]*[1  1 1  1;
%                                0  1 0 -1;
%                               -1  0 1  0;
%                                1 -1 1 -1]*rotor_speed_square

== matlab function xi3_flatness/Rigid Body Dynamics ==
  data: parameters input size=8; x_dot output size=12; u input size=4; x input size=12
function x_dot=fcn(parameters,u,x)
%% allocate inputs
m=parameters(1);
g=parameters(2);
M=diag([parameters(3) parameters(4) parameters(5)]);
f=u(1);
taub=u(2:4);
pn=x(1:3);
vn=x(4:6);
eta=x(7:9);
omegab=x(10:12);
%% define matrix Rbn , Lbn and Omega
phi=eta(1);
theta=eta(2);
psi=eta(3);
Rbn=[cos(theta)*cos(psi) sin(phi)*sin(theta)*cos(psi)-cos(phi)*sin(psi) cos(phi)*sin(theta)*cos(psi)+sin(phi)*sin(psi);
     cos(theta)*sin(psi) sin(phi)*sin(theta)*sin(psi)+cos(phi)*cos(psi) cos(phi)*sin(theta)*sin(psi)-sin(phi)*cos(psi);
     -sin(theta)         sin(phi)*cos(theta)                            cos(phi)*cos(theta)                           ];
Lbn=[1 sin(phi)*tan(theta) cos(phi)*tan(theta);
     0 cos(phi)            -sin(phi);
     0 sin(phi)/cos(theta) cos(phi)/cos(theta)];

%% nonlinear model: shown on the handout
pn_dot=vn;
vn_dot=1/m*Rbn*[0 0 f]'-[0 0 g]'; % -1/m*[Ax 0 0;0 Ay 0;0 0 Az]*pn_dot;    % pay attention to whether I need Ax, Ay, Az
eta_dot=Lbn*omegab;
omegab_dot=M\(taub-cross(omegab,M*omegab));
%% output x_dot
x_dot=[pn_dot;
       vn_dot;
       eta_dot;
       omegab_dot];
end
